simulink model "CAN_Model_v4bis"  (R2018b)
settings: Solver=VariableStepAuto  StartTime=0.0  StopTime=40  RelTol=1e-3
libraries: simulink_extras x1
(part 2 of 2)

== matlab function CAN_Model_v4bis/CanTrafficNode1/Receiver/MATLAB BusRxAndDestuff ==
  data: Bus input; EOF output; ACK output; Enable input; AckEnable input; Frame input; Index input; Error output; DeStuffedFrame output; NextFrame output; NextIndex output; Count input; NextCount output; Jump input; NextJump output
function [EOF, ACK, Error, DeStuffedFrame, NextFrame, NextIndex, NextCount, NextJump] = BusRxAndDestuff(Bus, Enable, AckEnable, Frame, Index, Count, Jump)

DeStuffedFrame = zeros(111,1);
NextCount = 0;
NextFrame = zeros(111,1);
EOF = 0;
Error = 0;
NextIndex = 1;
NextJump = 0;
ACK = 1;

if Enable == 1
    if Index <= 111
        NextFrame = Frame;
        if (Index <= 98) || (Count == 4)
            if (Index == 1) || (Jump == 1)
                NextFrame(Index) = Bus;
                NextIndex = Index + 1;
            else
                if Count == 4
                    NextIndex = Index;
                    NextCount = 0;
                    NextJump = 1;
                else
                    NextFrame(Index) = Bus;
                    NextIndex = Index + 1;
                    if Bus == NextFrame(Index - 1)
                        NextCount = Count + 1;
                    else
                        NextCount = 0;
                    end
                end
            end
        else
            if(Index == 99) && (AckEnable == 1)
                ACK = 0;
            end
            NextFrame(Index) = Bus;
            NextIndex = Index + 1;
        end
    else
        EOF = 1;
        DeStuffedFrame = Frame;
    end
end
end

== matlab function CAN_Model_v4bis/CanTrafficNode1/Transmitter/CAN_Transmission ==
  data: frame input; frame_length input; enable input; serial output; tx_completed output; index input; next_index output
function [serial,  tx_completed ,next_index]  = fcn(frame, frame_length, enable, index)

if enable == 1
    if index > frame_length
        serial = 1;
        tx_completed = 1;
        next_index = 1;
    else
        serial = frame(index);
        next_index = index + 1;
        tx_completed = 0;
    end
else
    tx_completed = 0;
    serial = 1;
    next_index = 1;
end

end

== matlab function CAN_Model_v4bis/CanTrafficNode1/Triggered Subsystem1/CAN Stuffer ==
  data: frame input; stuffed_frame output; stuffed_frame_length output
function [stuffed_frame, stuffed_frame_length] = CANstuffer(frame)

NumOfZeros = 0;
NumOfOnes = 0;
NumOfStuffedBits = 0;

stuffed_frame = zeros(135,1);

for i = 1 : length(frame)
    if frame(i) == 0
        NumOfZeros = NumOfZeros + 1;
        NumOfOnes = 0;
    else
        NumOfOnes = NumOfOnes + 1;
        NumOfZeros = 0;
    end
    
    if NumOfZeros == 5
        NumOfZeros = 0;
        NumOfOnes = NumOfOnes + 1;
        
        %Appending the stuffed ONE
        stuffed_frame(i + NumOfStuffedBits) = frame(i);
        NumOfStuffedBits = NumOfStuffedBits + 1;
        stuffed_frame(i + NumOfStuffedBits) = 1;
        
    elseif NumOfOnes == 5
        NumOfOnes = 0;
        NumOfZeros = NumOfZeros + 1;
        
        %Appending the stuffed ZERO
        stuffed_frame(i + NumOfStuffedBits) = frame(i);
        NumOfStuffedBits = NumOfStuffedBits + 1;
        stuffed_frame(i + NumOfStuffedBits) = 0;
        
    else
        stuffed_frame(i + NumOfStuffedBits) = frame(i); 
    end
end
stuffed_frame_length = length(frame) + NumOfStuffedBits;
end

== matlab function CAN_Model_v4bis/CanTrafficNode1/Triggered Subsystem1/MATLAB Function ==
  data: Init input; InitCmplt output; Bus input; index input; next_index output
function [InitCmplt, next_index] = BusIdleSensing(Init, Bus, index)

InitCmplt = 0;

if Init == 1
    if Bus == 1
        if index < 10 %Number of one to wait for EOF (after 11 ones)
            next_index = index + 1;
        else
            next_index = 0;
            InitCmplt = 1;
        end
    else
        next_index = 0;
    end
else
   next_index = 0;
end

end

== matlab function CAN_Model_v4bis/CanTrafficNode1/Triggered Subsystem1/MATLAB Function1 ==
  data: Bus input; SOF output; BusIdle input
function SOF = SOF_Detection(Bus, BusIdle)

if BusIdle == 1 %Checks the current state of the FSM
    if Bus == 0
        SOF = 1; %SOF Detected, the flag goes to One!
    else
        SOF = 0;    
    end
else
    SOF = 0;
end

end

== matlab function CAN_Model_v4bis/CanTrafficNode1/Triggered Subsystem1/MATLAB Function2 ==
  data: ArbCmplt output; Win output; Arbitration input; Bus input; ID input; ID_Lenght input; next_index output; index input
function [ArbCmplt, Win, next_index] = arbitration(Arbitration, Bus, ID, ID_Lenght, index)

ArbCmplt = 0;
Win = 0;
next_index = 1;

if Arbitration == 1
    if index <= ID_Lenght
        if ID(index) == Bus
            next_index = index + 1;
        else
            Win = 0;
            ArbCmplt = 1;
        end
    else
        next_index = 1;
        Win = 1;
        ArbCmplt = 1;
    end    
    
else next_index = 1;
    
end
end

== matlab function CAN_Model_v4bis/MATLAB Function1 ==
  data: ID output
function ID = randomID2()

%if EOF == 1
    ID = [randi([0, 1], 1, 11)];
%else
   % ID = initialID;
%end

end
